simulink library "rtsync_lib"  (Simulink 7.1)
undefined symbols (not defined in the file): Ts
settings Model: Creator=henrik  LastModifiedBy=henrik  ExtModeAutoUpdateStatusClock=off

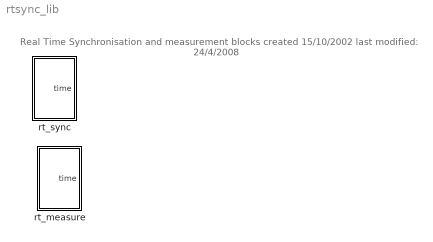
== system rtsync_lib ==
  note: Real Time Synchronisation and
      | measurement blocks
      | created 15/10/2002
      | last modified: 24/4/2008
  rt_measure : Subsystem  mask{Ts=Ts, strict=off, outflag=on}
      mask prompts: Ts "Sample Time"; strict "Strict Sample time"; outflag "Enable output"
      mask help:
      | Real time measurement block.
      | Parameter: Ts = discrete sample time
      | output: actual time between samples.
      mask init:
      | load_system simulink
      | %---------------------------------------------------------------------------
      | % Ts Output
      | block = 'time';
      | system_block = [gcb '/' block];
      | srcblock= 'S-Function';
      | system_srcblock= [gcb '/' srcblock];
      | pos=get_param(system_block,'position');
      | blocktype=get_param(system_block,'blocktype');
      | % Check the value selected 
      | % Get the mask parameter values. This is a cell array of strings.
      | maskStr = get_param(gcb,'MaskValues');
      | % The outflag is the 3rd mask parameter.
      | if strcmp(maskStr{3},'on'),
      |     if ~strcmp(blocktype,'Outport')
      |         delete_line(gcb, [srcblock '/1'], [block '/1']);
      |         delete_block(system_block);
      |         add_block('simulink/Sinks/Out1',system_block,'position',pos);
      |         add_line(gcb, [srcblock '/1'], [block '/1']);
      |     end
      | else
      |     if ~strcmp(blocktype,'Terminator')
      |         delete_line(gcb, [srcblock '/1'], [block '/1']);
      |         delete_block(system_block);
      |         add_block('simulink/Sinks/Terminator',system_block,'position',pos);
      |         add_line(gcb, [srcblock '/1'], [block '/1']);
      |     end
      | end
      mask Display: fprintf('Real\n Time\n measure')
  rt_sync : Subsystem  mask{Ts=Ts, strict=off, outflag=on}
      mask prompts: Ts "Sample Time"; strict "Strict Sample time"; outflag "Enable output"
      mask help:
      | Real time synchronisation block.
      | Parameter: Ts = discrete sample time
      | optional output: actual time between samples.
      mask init: same as rtsync_lib/rt_measure
      mask Display: fprintf('Real\n Time\n sync')

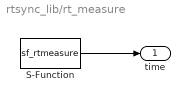
== system rtsync_lib/rt_measure ==
  S-Function : S-Function  FunctionName=sf_rtmeasure  Parameters=Ts,strict  EnableBusSupport=off
  time : Outport  OutDataType=sfix(16)  OutScaling=2^0
  wires:
  S-Function/1 -> time/1

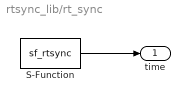
== system rtsync_lib/rt_sync ==
  S-Function : S-Function  FunctionName=sf_rtsync  Parameters=Ts,strict  EnableBusSupport=off
  time : Outport  OutDataType=sfix(16)  OutScaling=2^0
  wires:
  S-Function/1 -> time/1
